simulink model "Iterative_Learning_Control"  (R2021b)
settings: Solver=VariableStepAuto  StartTime=0.0  StopTime=15  RelTol=1e-3
undefined symbols (not defined in the file): gamma, Kd, Kp, q_d, q_dq_init
settings Model: Creator=Yafei Ou  LastModifiedBy=Kirill

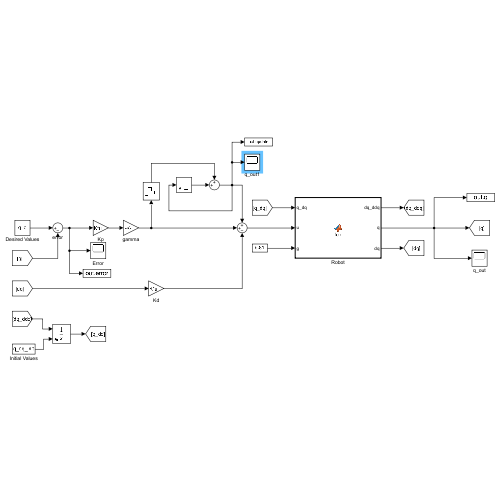
[thumbnail: Simulink's stored preview of the top-level diagram]
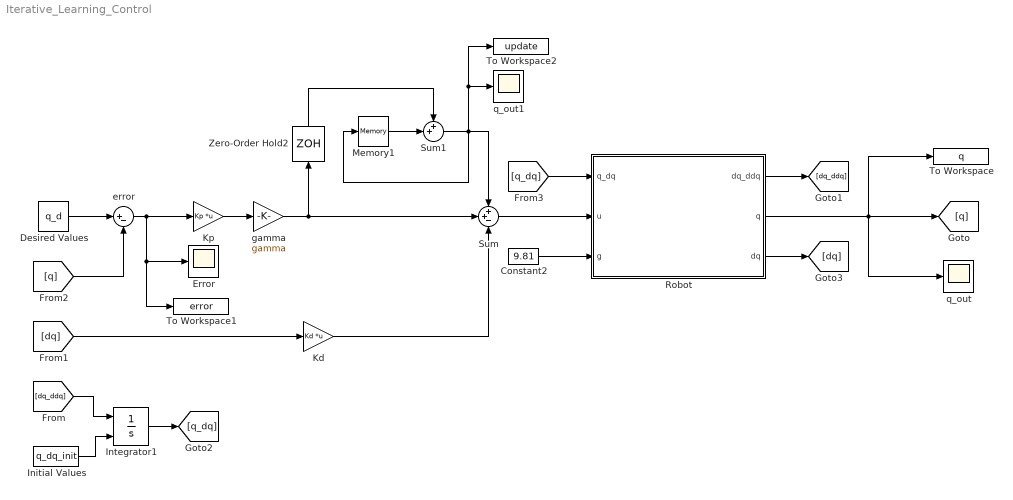
== system Iterative_Learning_Control ==
  Constant2 : Constant  Value=9.81
  Desired Values : Constant  Value=q_d
  Error : Scope
  Initial Values : Constant  Value=q_dq_init
  Integrator1 : Integrator  InitialConditionSource=external
  Kd : Gain  Gain=Kd  Multiplication=Matrix(K*u)
  Kp : Gain  Gain=Kp  Multiplication=Matrix(K*u)
  Memory1 : Memory  InheritSampleTime=on
  Robot : MATLAB Function  TreatAsAtomicUnit=on
  Sum : Sum  Inputs=++-
  Sum1 : Sum  Inputs=++|
  To Workspace : ToWorkspace  VariableName=q  SampleTime=-1
  To Workspace1 : ToWorkspace  VariableName=error  SampleTime=-1
  To Workspace2 : ToWorkspace  VariableName=update  SampleTime=-1
  Zero-Order Hold2 : ZeroOrderHold  SampleTime=2
  error : Sum  Inputs=|+-
  gamma : Gain  Gain=gamma
  q_out : Scope
  q_out1 : Scope
  wires:
  Desired Values/1 -> error/1
  Kp/1 -> gamma/1
  Kd/1 -> Sum/3
  Memory1/1 -> Sum1/2
  gamma/1 -> Zero-Order Hold2/1, Sum/2
  Sum1/1 -> Memory1/1, To Workspace2/1, q_out1/1, Sum/1
  Robot/2(q) -> To Workspace/1, q_out/1, [q]
  Zero-Order Hold2/1 -> Sum1/1
  error/1 -> To Workspace1/1, Error/1, Kp/1
  Constant2/1 -> Robot/3(g)
  Robot/1(dq_ddq) -> [dq_ddq]
  Initial Values/1 -> Integrator1/2
  [dq_ddq] -> Integrator1/1
  Integrator1/1 -> [q_dq]
  Robot/3(dq) -> [dq]
  [dq] -> Kd/1
  [q] -> error/2
  Sum/1 -> Robot/2(u)
  [q_dq] -> Robot/1(q_dq)

== matlab function Iterative_Learning_Control/Robot ==
  data: q_dq input; dq_ddq output; u input; q output; dq output; g input
function [dq_ddq,q,dq] = fcn(q_dq,u,g)
    q = q_dq(1:length(q_dq)/2);
    dq = q_dq(length(q_dq)/2+1:length(q_dq));
    g_num = g;


    M = M_fun(q);
    C = C_fun(q,dq);
    G = G_fun(q,g_num);

    ddq = M\(u - C - G);
    
    dq_ddq = [dq;ddq];

end
